simulink model "wrist_flexion"  (Simulink 6.6)
settings: Solver=ode3  SolverMode=SingleTasking  StartTime=0.0  StopTime=Inf  FixedStep=.001  RelTol=1e-3
libraries: xpclib x10, xpcnilib x4, simulink x3, limblab x3, dsparch4 x2, xpcmeasurementcomputinglib x2, dspsigops x2, IntelSMIlibR2007b x1
settings Model: Creator=Selket  LastModifiedBy=limblab  ExtModeArmWhenConnect=off  BufferReuse=off  ProdHWDeviceType=Generic->32-bit x86 compatible
settings OptimizationCC: BlockReduction=off  OptimizeBlockIOStorage=off  BufferReuse=off  ExpressionFolding=off  FoldNonRolledExpr=off  LocalBlockOutputs=off
settings DebuggingCC: MultiTaskCondExecSysMsg=none  StrictBusMsg=None
settings HardwareCC: ProdIntDivRoundTo=Zero  ProdEndianess=LittleEndian  ProdHWDeviceType=Generic->32-bit x86 compatible
settings RTWCC: SystemTargetFile=xpctarget.tlc  TemplateMakefile=xpc_default_tmf  Description=xPC Target  ProcessScript=xpctarget_make_rtw_hook  IncludeERTFirstTime=on
settings xpcTargetCC: TargetFcnLib=ansi_tfl_tmw.mat  GenFloatMathFcnCalls=ANSI_C  PortableWordSizes=off  xPCisDownloadable=off  xPCisDefaultEnv=off

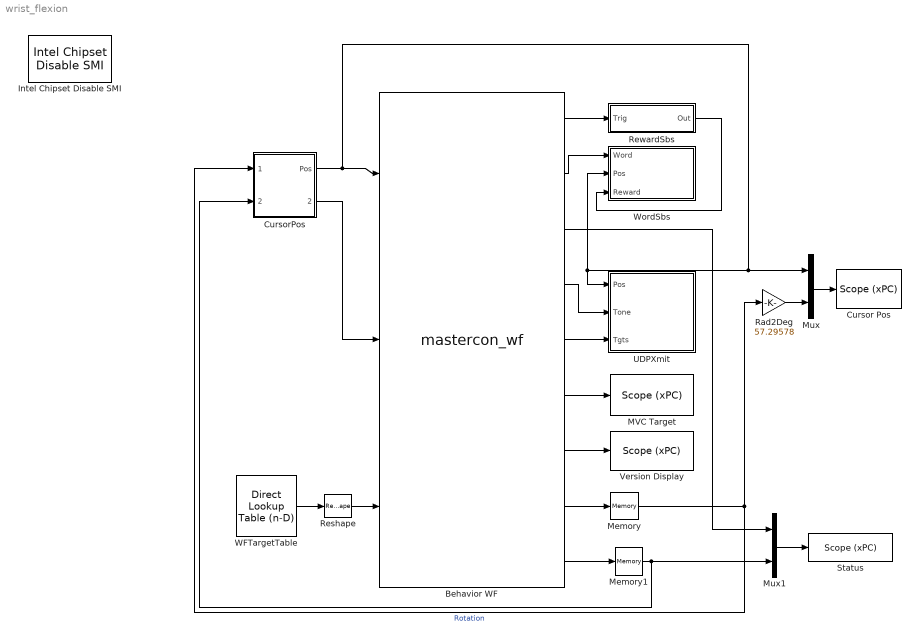
== system wrist_flexion ==
  Behavior WF : S-Function  FunctionName=mastercon_wf  Parameters=8 5 .5 .5 1 0 0 3 3 2 0 0 0 0 0 0 0 0.7854 0 .5 0
      mask Display:
      | disp('Master Control\nWrist-Flexion')
      | port_label('input',1,'cursor')
      | port_label('input',2,'cursor offset')
      | port_label('input',3,'target list')
      | port_label('output',1,'Reward')
      | port_label('output',2,'Word')
      | port_label('output',3,'Status')
      | port_label('output',4,'Tone')
      | port_label('output',5,'Targets')
      | port_label('output',6,'MVC Target')
      | port_label('output',7,'version')
      | port_label('output',8,'rotation')
      | port_label('output',9,'neural control flag')
  Cursor Pos : xpclib/Misc./Scope (xPC)   SystemSampleTime=-1  scopeno=2  scopetype=Target  autostart=on  viewmode=Numerical  formatstr="' X: %4.6f   , Y: %4.6f   , (Rotated %6.2f degrees)  '"  grid=on  ylimits=[-10,10]  nosamples=10  noprepostsamples=0  interleave=10  triggermode=FreeRun  triggersignal=1  triggerlevel=0.0  triggerslope=Either  triggerscope=1  triggersample=0  filename=data.dat  mode=Lazy  writesize=512  autorestart=off
  CursorPos : Subsystem
  Intel Chipset Disable SMI : IntelSMIlibR2007b/Intel Chipset Disable SMI
  MVC Target : xpclib/Misc./Scope (xPC)   SystemSampleTime=-1  scopeno=6  scopetype=Target  autostart=on  viewmode=Numerical  formatstr="' Quad 1: %6.4f X  , Quad 1: %6.4f Y  , Quad 2: %6.4f X  , Quad 2: %6.4f Y  , Quad 3: %6.4f X  , Quad 3: %6.4f Y  , Quad 4: %6.4f X  , Quad 4: %6.4f Y  '"  grid=on  ylimits=[-10,10]  nosamples=10  noprepostsamples=0  interleave=10  triggermode=FreeRun  triggersignal=1  triggerlevel=0.0  triggerslope=Either  triggerscope=1  triggersample=0  filename=data.dat  mode=Lazy  writesize=512  autorestart=off
  Memory : Memory  InheritSampleTime=on
  Memory1 : Memory  InheritSampleTime=on
  Mux : Mux  Inputs=2
  Mux1 : Mux  Inputs=2
  Rad2Deg : Gain  Gain=57.29578
  Reshape : Reshape  OutputDimensionality=Column vector (2-D)
  RewardSbs : Subsystem
  Status : xpclib/Misc./Scope (xPC)   SystemSampleTime=-1  scopeno=1  scopetype=Target  autostart=on  viewmode=Numerical  formatstr='%6.0f State,%6.0f Rewards,%6.0f Aborts,%6.0f Failures,%6.0f NeuralFlag'  grid=on  ylimits=[-10,10]  nosamples=10  noprepostsamples=0  interleave=10  triggermode=FreeRun  triggersignal=1  triggerlevel=0.0  triggerslope=Either  triggerscope=1  triggersample=0  filename=data.dat  mode=Lazy  writesize=512  autorestart=off
  UDPXmit : Subsystem
  Version Display : xpclib/Misc./Scope (xPC)   SystemSampleTime=-1  scopeno=4  scopetype=Target  autostart=on  viewmode=Numerical  formatstr='%6.0f major,%6.0f minor,%6.0f revision,%6.0f build'  grid=on  ylimits=[-10,10]  nosamples=10  noprepostsamples=0  interleave=10  triggermode=FreeRun  triggersignal=1  triggerlevel=0.0  triggerslope=Either  triggerscope=1  triggersample=0  filename=data.dat  mode=Lazy  writesize=512  autorestart=off
  WFTargetTable : simulink/Lookup Tables/Direct Lookup Table (n-D)  maskTabDims=2  explicitNumDims=1  outDims=2-D Matrix  tabIsInput=off  mxTable=[5 5 5 5 5 5 5 5 5 5 5 5 5 5 5 5;5 5 5 5 5 5 5 5 5 5 5 5 5 5 5 5;5 5 5 5 5 5 5 5 5 5 5 5 5 5 5 5;5 5 5 5 5 5 5 5 5 5 5 5 5 5 5 5;0 0 0 0 0 0 0 0 0 0 0 0 0 0 0 0;0 0 0 0 0 0 0 0 0 0 0 0 0 0 0 0]  clipFlag=Warning  samptime=0.001
  WordSbs : Subsystem
  wires:
  Behavior WF/2 -> WordSbs/1(Word)
  Behavior WF/1 -> RewardSbs/1(Trig)
  Behavior WF/4 -> UDPXmit/2(Tone)
  Behavior WF/5 -> UDPXmit/3(Tgts)
  CursorPos/1(Pos) -> Behavior WF/1, Mux/1, UDPXmit/1(Pos), WordSbs/2(Pos)
  Mux/1 -> Cursor Pos/1
  Rad2Deg/1 -> Mux/2
  RewardSbs/1(Out) -> WordSbs/3(Reward)
  Memory/1 -> Rad2Deg/1, CursorPos/1(Rotation)  "Rotation"
  WFTargetTable/1 -> Reshape/1
  Behavior WF/8 -> Memory/1
  Behavior WF/7 -> Version Display/1
  Behavior WF/6 -> MVC Target/1
  Reshape/1 -> Behavior WF/3
  CursorPos/2(Offsets) -> Behavior WF/2
  Behavior WF/9 -> Memory1/1
  Memory1/1 -> CursorPos/2(Neural control flag), Mux1/2
  Behavior WF/3 -> Mux1/1
  Mux1/1 -> Status/1

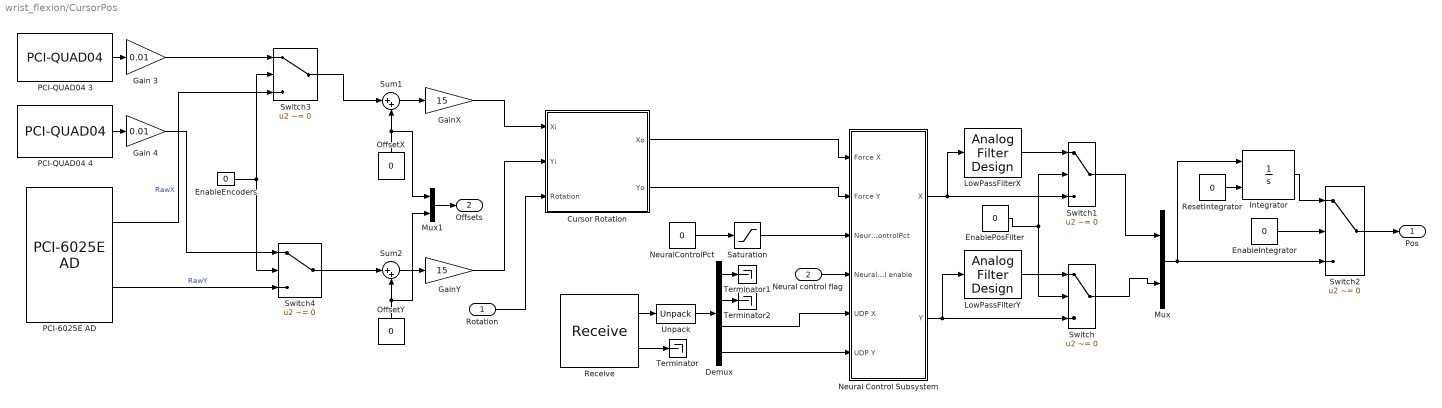
== system wrist_flexion/CursorPos ==
  Rotation : Inport
  Neural control flag : Inport  Port=2
  Cursor Rotation : Subsystem
  Demux : Demux
  EnableEncoders : Constant  Value=0
  EnableIntegrator : Constant  Value=0
  EnablePosFilter : Constant  Value=0
  Gain 3 : Gain  Gain=0.01
  Gain 4 : Gain  Gain=0.01
  GainX : Gain  Gain=15
  GainY : Gain  Gain=15
  Integrator : Integrator  ExternalReset=rising  LimitOutput=on  UpperSaturationLimit=15  LowerSaturationLimit=-15
  LowPassFilterX : dsparch4/Analog Filter Design  method=Butterworth  filttype=Lowpass  N=8  Wlo=15  Whi=80  Rp=2  Rs=40
  LowPassFilterY : dsparch4/Analog Filter Design  method=Butterworth  filttype=Lowpass  N=8  Wlo=15  Whi=80  Rp=2  Rs=40
  Mux : Mux  Inputs=2
  Mux1 : Mux  Inputs=2
  Neural Control Subsystem : Subsystem
  NeuralControlPct : Constant  Value=0
  OffsetX : Constant  Orientation=up  Value=0
  OffsetY : Constant  Orientation=up  Value=0
  PCI-6025E AD : xpcnilib/A//D/PCI-6025E AD  channel=[9 10]  range=[-10]  coupling=[0]  sampletime=0.001  slot=-1
  PCI-QUAD04 3 : xpcmeasurementcomputinglib/Incremental Encoder/PCI-QUAD04   channel=3  resetmode=on  polarity=Positive Index  mode=Normal  limit=0  range=-2^23...+2^23-1  speed=1x  prescale=0  ts=0.001  convbaseaddr=-1
  PCI-QUAD04 4 : xpcmeasurementcomputinglib/Incremental Encoder/PCI-QUAD04   channel=4  resetmode=on  polarity=Positive Index  mode=Normal  limit=0  range=-2^23...+2^23-1  speed=1x  prescale=0  ts=0.001  convbaseaddr=-1
  Receive : xpclib/UDP/Receive  ipAddress=0.0.0.0  ipPort=24999  width=16  sampletime=0.01
  ResetIntegrator : Constant  Value=0
  Saturation : Saturate  UpperLimit=100  LowerLimit=0
  Sum1 : Sum  Inputs=|++
  Sum2 : Sum  Inputs=|++
  Switch{,1..4} (5 alike) : Switch  Criteria=u2 ~= 0
  Terminator : Terminator
  Terminator1 : Terminator
  Terminator2 : Terminator
  Unpack : xpclib/UDP/Unpack  dimensions={[1,4]}  datatypes={'single'}  byteAlign=1
  Pos : Outport
  Offsets : Outport  Port=2
  wires:
  Rotation/1 -> Cursor Rotation/3(Rotation)
  OffsetX/1 -> Sum1/2, Mux1/1
  OffsetY/1 -> Sum2/2, Mux1/2
  Mux1/1 -> Offsets/1
  PCI-QUAD04 4/1 -> Gain 4/1
  PCI-QUAD04 3/1 -> Gain 3/1
  PCI-6025E AD/1 -> Switch3/3  "RawX"
  PCI-6025E AD/2 -> Switch4/3  "RawY"
  Gain 4/1 -> Switch4/1
  Gain 3/1 -> Switch3/1
  Sum2/1 -> GainY/1
  Sum1/1 -> GainX/1
  Switch3/1 -> Sum1/1
  Switch4/1 -> Sum2/1
  EnableEncoders/1 -> Switch3/2, Switch4/2
  Receive/1 -> Unpack/1
  Receive/2 -> Terminator/1
  Unpack/1 -> Demux/1
  Demux/1 -> Terminator1/1
  NeuralControlPct/1 -> Saturation/1
  Saturation/1 -> Neural Control Subsystem/3(NeuralControlPct)
  Cursor Rotation/1(Xo) -> Neural Control Subsystem/1(Force X)
  Cursor Rotation/2(Yo) -> Neural Control Subsystem/2(Force Y)
  EnableIntegrator/1 -> Switch2/2
  Mux/1 -> Switch2/3, Integrator/1
  Integrator/1 -> Switch2/1
  ResetIntegrator/1 -> Integrator/2
  Switch2/1 -> Pos/1
  Demux/3 -> Neural Control Subsystem/5(UDP X)
  Demux/4 -> Neural Control Subsystem/6(UDP Y)
  Demux/2 -> Terminator2/1
  Neural control flag/1 -> Neural Control Subsystem/4(Neural control enable)
  LowPassFilterX/1 -> Switch1/1
  LowPassFilterY/1 -> Switch/1
  EnablePosFilter/1 -> Switch/2, Switch1/2
  Neural Control Subsystem/1(X) -> Switch1/3, LowPassFilterX/1
  Neural Control Subsystem/2(Y) -> Switch/3, LowPassFilterY/1
  Switch1/1 -> Mux/1
  Switch/1 -> Mux/2
  GainY/1 -> Cursor Rotation/2(Yi)
  GainX/1 -> Cursor Rotation/1(Xi)

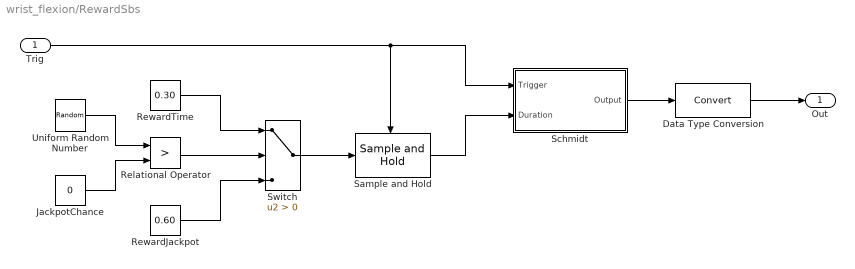
== system wrist_flexion/RewardSbs ==
  Trig : Inport
  Data Type Conversion : DataTypeConversion
  JackpotChance : Constant  Value=0
  Relational Operator : RelationalOperator  Operator=>  LogicOutDataTypeMode=Boolean
  RewardJackpot : Constant  Value=0.60
  RewardTime : Constant  Value=0.30
  Sample and Hold : dspsigops/Sample and Hold  SystemSampleTime=-1  trig=Rising edge  initCond=0  latchinput=off
  Schmidt : Subsystem
  Switch : Switch  Criteria=u2 > Threshold  ZeroCross=off
  Uniform Random Number : UniformRandomNumber  Minimum=0  Maximum=100  SampleTime=0.001
  Out : Outport
  wires:
  Trig/1 -> Schmidt/1(Trigger), Sample and Hold/Trigger
  Data Type Conversion/1 -> Out/1
  Schmidt/1(Output) -> Data Type Conversion/1
  Sample and Hold/1 -> Schmidt/2(Duration)
  RewardTime/1 -> Switch/1
  RewardJackpot/1 -> Switch/3
  Switch/1 -> Sample and Hold/1
  Uniform Random Number/1 -> Relational Operator/1
  Relational Operator/1 -> Switch/2
  JackpotChance/1 -> Relational Operator/2

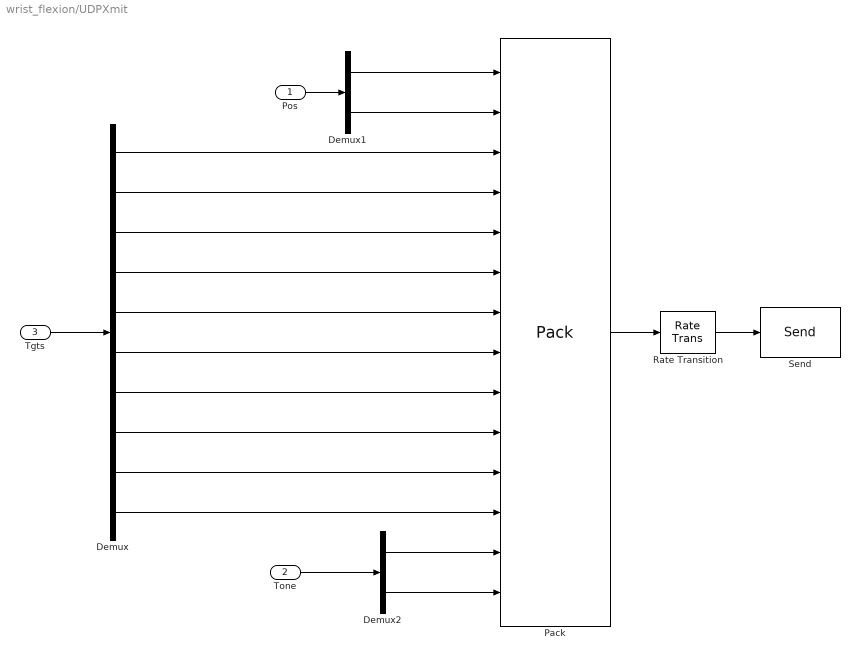
== system wrist_flexion/UDPXmit ==
  Pos : Inport
  Tone : Inport  Port=2
  Tgts : Inport  Port=3
  Demux : Demux  Outputs=10
  Demux1 : Demux  Outputs=2
  Demux2 : Demux  Outputs=2
  Pack : xpclib/UDP/Pack  datatypes={'double', 'double','double','double','double','double','double','double','double','double','double','double','double','double'}  byteAlign=1
  Rate Transition : RateTransition
  Send : xpclib/UDP/Send  ipAddress=192.168.0.2  ipPort=25000  localPort=-1  sampletime=.02
  wires:
  Rate Transition/1 -> Send/1
  Pack/1 -> Rate Transition/1
  Demux/10 -> Pack/12
  Demux/9 -> Pack/11
  Demux/8 -> Pack/10
  Demux/7 -> Pack/9
  Demux/6 -> Pack/8
  Demux/5 -> Pack/7
  Demux/4 -> Pack/6
  Demux/3 -> Pack/5
  Demux/2 -> Pack/4
  Demux/1 -> Pack/3
  Demux1/1 -> Pack/1
  Demux1/2 -> Pack/2
  Pos/1 -> Demux1/1
  Demux2/1 -> Pack/13
  Demux2/2 -> Pack/14
  Tone/1 -> Demux2/1
  Tgts/1 -> Demux/1

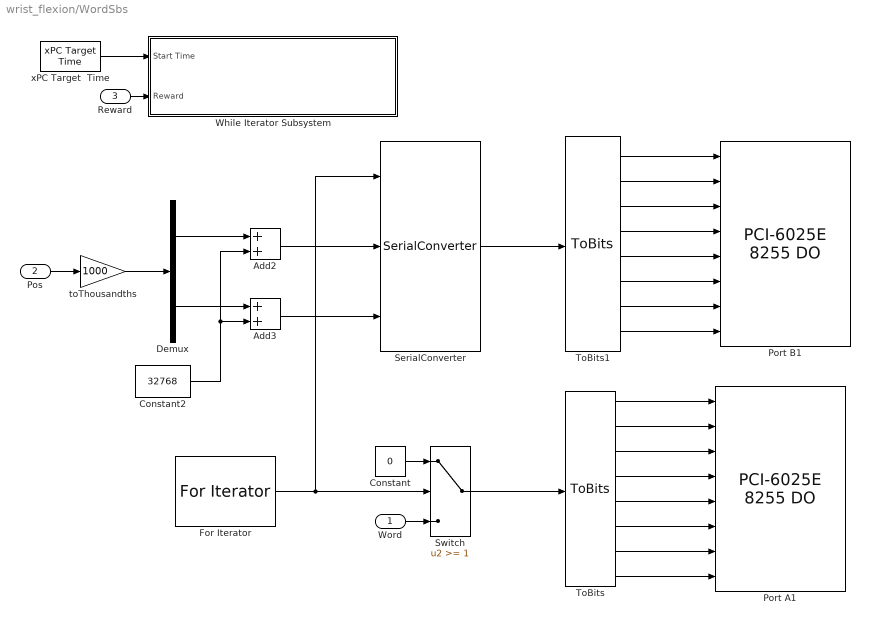
== system wrist_flexion/WordSbs ==
  Word : Inport
  Pos : Inport  Port=2
  Reward : Inport  Port=3
  Add2 : Sum  OutScaling=2^-10
  Add3 : Sum  OutScaling=2^-10
  Constant : Constant  Value=0
  Constant2 : Constant  Value=32768
  Demux : Demux  Outputs=2
  For Iterator : ForIterator  IterationLimit=4  IndexMode=Zero-based  IterationVariableDataType=double
  Port A1 : xpcnilib/Digital Output/PCI-6025E 8255 DO  channel=1:8  port=A  reset=[1]  initValue=[0]  chip=1  sampletime=-1  slot=-1
  Port B1 : xpcnilib/Digital Output/PCI-6025E 8255 DO  channel=1:8  port=B  reset=[1]  initValue=[0]  chip=1  sampletime=-1  slot=-1
  SerialConverter : limblab/SerialConverter
  Switch : Switch  Threshold=1  ZeroCross=off
  ToBits : limblab/ToBits
  ToBits1 : limblab/ToBits
  While Iterator Subsystem : Subsystem  TreatAsAtomicUnit=on
  toThousandths : Gain  Gain=1000
  "xPC Target  Time " : xpclib/Misc./xPC Target  Time   ts=-1
  wires:
  ToBits/1 -> Port A1/1
  ToBits/2 -> Port A1/2
  ToBits/3 -> Port A1/3
  ToBits/4 -> Port A1/4
  ToBits/5 -> Port A1/5
  ToBits/6 -> Port A1/6
  ToBits/7 -> Port A1/7
  ToBits/8 -> Port A1/8
  Switch/1 -> ToBits/1
  For Iterator/1 -> Switch/2, SerialConverter/1
  "xPC Target  Time "/1 -> While Iterator Subsystem/1(Start Time)
  Constant/1 -> Switch/1
  Constant2/1 -> Add2/2, Add3/2
  ToBits1/8 -> Port B1/8
  ToBits1/7 -> Port B1/7
  ToBits1/6 -> Port B1/6
  ToBits1/5 -> Port B1/5
  ToBits1/1 -> Port B1/1
  ToBits1/2 -> Port B1/2
  ToBits1/3 -> Port B1/3
  ToBits1/4 -> Port B1/4
  SerialConverter/1 -> ToBits1/1
  Word/1 -> Switch/3
  Add2/1 -> SerialConverter/2
  Add3/1 -> SerialConverter/3
  Pos/1 -> toThousandths/1
  Demux/1 -> Add2/1
  Demux/2 -> Add3/1
  toThousandths/1 -> Demux/1
  Reward/1 -> While Iterator Subsystem/2(Reward)

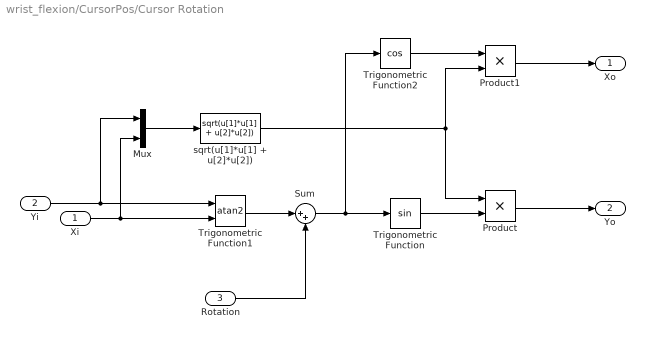
== system wrist_flexion/CursorPos/Cursor Rotation ==
  Xi : Inport
  Yi : Inport  Port=2
  Rotation : Inport  Port=3
  Mux : Mux  Inputs=2
  Product : Product  RndMeth=Zero
  Product1 : Product  RndMeth=Zero
  Sum : Sum  Inputs=|++
  Trigonometric Function : Trigonometry
  Trigonometric Function1 : Trigonometry  Operator=atan2
  Trigonometric Function2 : Trigonometry  Operator=cos
  sqrt(u[1]*u[1] + u[2]*u[2]) : Fcn  Expr=sqrt(u[1]*u[1] + u[2]*u[2])
  Xo : Outport
  Yo : Outport  Port=2
  wires:
  Rotation/1 -> Sum/2
  Trigonometric Function1/1 -> Sum/1
  Yi/1 -> Trigonometric Function1/1, Mux/1
  Xi/1 -> Trigonometric Function1/2, Mux/2
  Mux/1 -> sqrt(u[1]*u[1] + u[2]*u[2])/1
  Trigonometric Function/1 -> Product/2
  Product/1 -> Yo/1
  sqrt(u[1]*u[1] + u[2]*u[2])/1 -> Product/1, Product1/2
  Sum/1 -> Trigonometric Function/1, Trigonometric Function2/1
  Product1/1 -> Xo/1
  Trigonometric Function2/1 -> Product1/1

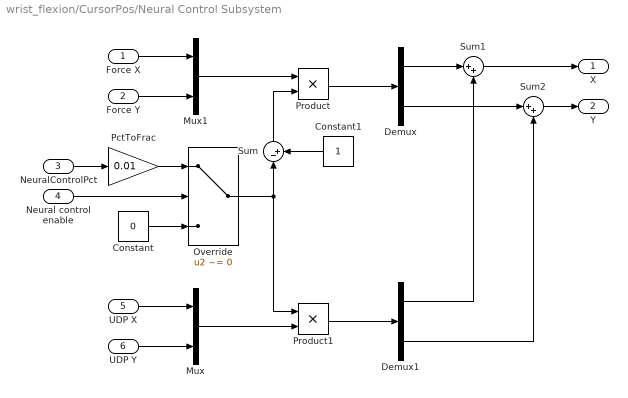
== system wrist_flexion/CursorPos/Neural Control Subsystem ==
  Force X : Inport
  Force Y : Inport  Port=2
  NeuralControlPct : Inport  Port=3
  Neural control enable : Inport  Port=4
  UDP X : Inport  Port=5
  UDP Y : Inport  Port=6
  Constant : Constant  Value=0
  Constant1 : Constant  Orientation=left
  Demux : Demux  Outputs=2
  Demux1 : Demux  Outputs=2
  Mux : Mux  Inputs=2
  Mux1 : Mux  Inputs=2
  Override : Switch  Criteria=u2 ~= 0  ZeroCross=off
  PctToFrac : Gain  Gain=0.01
  Product : Product  RndMeth=Zero
  Product1 : Product  RndMeth=Zero
  Sum : Sum  Orientation=up  Inputs=|-+
  Sum1 : Sum  Inputs=|++
  Sum2 : Sum  Inputs=|++
  X : Outport
  Y : Outport  Port=2
  wires:
  NeuralControlPct/1 -> PctToFrac/1
  UDP X/1 -> Mux/1
  UDP Y/1 -> Mux/2
  Neural control enable/1 -> Override/2
  Force X/1 -> Mux1/1
  Force Y/1 -> Mux1/2
  Mux/1 -> Product1/2
  Mux1/1 -> Product/1
  Constant1/1 -> Sum/2
  Override/1 -> Sum/1, Product1/1
  Sum/1 -> Product/2
  Product/1 -> Demux/1
  Product1/1 -> Demux1/1
  Demux/1 -> Sum1/1
  Sum1/1 -> X/1
  Demux/2 -> Sum2/1
  Sum2/1 -> Y/1
  Demux1/1 -> Sum1/2
  Demux1/2 -> Sum2/2
  Constant/1 -> Override/3
  PctToFrac/1 -> Override/1

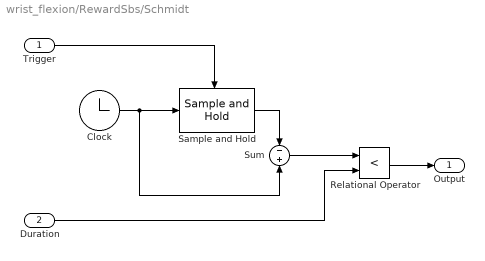
== system wrist_flexion/RewardSbs/Schmidt ==
  Trigger : Inport
  Duration : Inport  Port=2
  Clock : Clock
  Relational Operator : RelationalOperator  Operator=<  LogicOutDataTypeMode=Boolean
  Sample and Hold : dspsigops/Sample and Hold  SystemSampleTime=-1  trig=Rising edge  initCond=-1000  latchinput=off
  Sum : Sum  Inputs=-+
  Output : Outport
  wires:
  Clock/1 -> Sum/2, Sample and Hold/1
  Sample and Hold/1 -> Sum/1
  Sum/1 -> Relational Operator/1
  Duration/1 -> Relational Operator/2
  Relational Operator/1 -> Output/1
  Trigger/1 -> Sample and Hold/Trigger

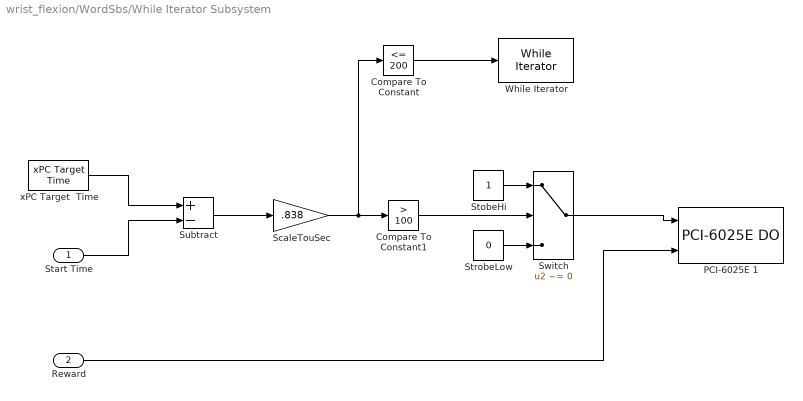
== system wrist_flexion/WordSbs/While Iterator Subsystem ==
  Start Time : Inport
  Reward : Inport  Port=2
  Compare To Constant : simulink/Logic and Bit Operations/Compare To Constant  SystemSampleTime=-1  relop=<=  const=200  LogicOutDataTypeMode=boolean
  Compare To Constant1 : simulink/Logic and Bit Operations/Compare To Constant  SystemSampleTime=-1  relop=>  const=100  LogicOutDataTypeMode=boolean  ZeroCross=off
  PCI-6025E 1 : xpcnilib/Digital Output/PCI-6025E DO  channel=[1 2]  reset=[1]  initValue=[0]  sampletime=-1  slot=-1
  ScaleTouSec : Gain  Gain=.838
  StobeHi : Constant
  StrobeLow : Constant  Value=0
  Subtract : Sum  Inputs=+-  OutScaling=2^-10
  Switch : Switch  Criteria=u2 ~= 0
  While Iterator : WhileIterator  MaxIters=-1  WhileBlockType=do-while
  "xPC Target  Time " : xpclib/Misc./xPC Target  Time   ts=-1
  wires:
  "xPC Target  Time "/1 -> Subtract/1
  Start Time/1 -> Subtract/2
  Subtract/1 -> ScaleTouSec/1
  Compare To Constant/1 -> While Iterator/1
  ScaleTouSec/1 -> Compare To Constant/1, Compare To Constant1/1
  Compare To Constant1/1 -> Switch/2
  StobeHi/1 -> Switch/1
  StrobeLow/1 -> Switch/3
  Switch/1 -> PCI-6025E 1/1
  Reward/1 -> PCI-6025E 1/2
